simulink model "chap3_2sim"  (Simulink 6.3)
settings: Solver=ode45  StartTime=0.0  StopTime=10.0  RelTol=1e-3
libraries: simulink x1, simulink_extras x1
settings Model: Creator=hp  LastModifiedBy=Administrator  ExtModeTrigMode=oneshot  ExtModeArmWhenConnect=off
settings DataIOCC: LimitDataPoints=off
settings OptimizationCC: BlockReduction=off  BooleanDataType=off
settings DebuggingCC: SolverPrmCheckMsg=none
settings HardwareCC: TargetUnknown=on

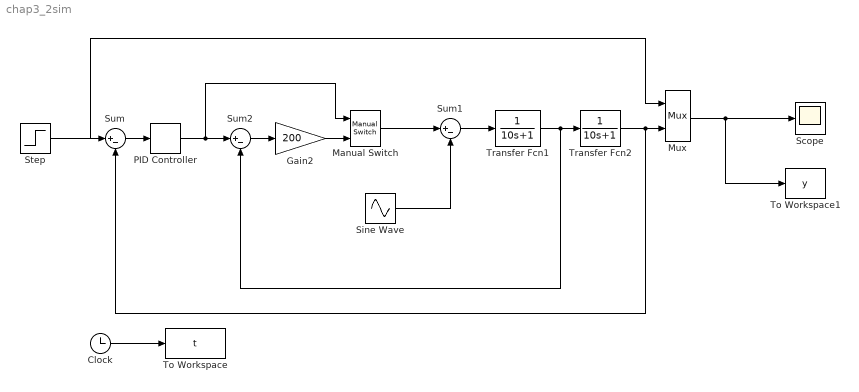
== system chap3_2sim ==
  Clock : Clock
      settings: Decimation=10
  Gain2 : Gain  Gain=200  SaturateOnIntegerOverflow=on
  Manual Switch : simulink/Signal Routing/Manual Switch  sw=1  action=0
  Mux : Mux  Inputs=2
  PID Controller : simulink_extras/Additional Linear/PID Controller  P=50  I=5  D=0
  Scope : Scope
      settings: YMin=-0.1  YMax=1
  Sine Wave : Sin  Frequency=50  SampleTime=0
  Step : Step  Time=0  SampleTime=0
  Sum : Sum  Inputs=|+-  SaturateOnIntegerOverflow=on  InputSameDT=on
  Sum1 : Sum  Inputs=|+-  SaturateOnIntegerOverflow=on  InputSameDT=on
  Sum2 : Sum  Inputs=|+-  SaturateOnIntegerOverflow=on  InputSameDT=on
  To Workspace : ToWorkspace  VariableName=t  SampleTime=-1  SaveFormat=Array
  To Workspace1 : ToWorkspace  VariableName=y  SampleTime=-1  SaveFormat=Array
  Transfer Fcn1 : TransferFcn  Denominator=[10 1]
  Transfer Fcn2 : TransferFcn  Denominator=[10 1]
  wires:
  Mux/1 -> Scope/1, To Workspace1/1
  Sum/1 -> PID Controller/1
  Step/1 -> Sum/1, Mux/1
  Sine Wave/1 -> Sum1/2
  Gain2/1 -> Manual Switch/2
  PID Controller/1 -> Manual Switch/1, Sum2/1
  Transfer Fcn1/1 -> Sum2/2, Transfer Fcn2/1
  Transfer Fcn2/1 -> Mux/2, Sum/2
  Sum2/1 -> Gain2/1
  Clock/1 -> To Workspace/1
  Sum1/1 -> Transfer Fcn1/1
  Manual Switch/1 -> Sum1/1
